simulink model "DisplayModel_Step3_done"  (R2013b)
settings: Solver=FixedStepDiscrete  StartTime=0.0  StopTime=10.0  FixedStep=0.2  RelTol=1e-3
undefined symbols (not defined in the file): sldvsubsys
libraries: simulink x6, sldvlib x3
settings Model: CovPath=LandingGearModes  CovMetricSettings=dcmw  CovHTMLOptions=-sRT=1 -aTS=1 -bRG=1 -bTC=1 -hTR=0 -nFC=0 -scm=1 -bcm=1 -xEv=0  CovModelRefEnable=off  Creator=siddhars  LastModifiedBy=rruff
settings OptimizationCC: InlineParams=on  ExpressionDepthLimit=2147483647  OptimizeModelRefInitCode=on  LifeSpan=1
settings DebuggingCC: StateNameClashWarn=warning
settings RTWCC: SystemTargetFile=ert.tlc  TemplateMakefile=ert_default_tmf  Description=Embedded Coder  ProcessScript=ert_make_rtw_hook  PortableWordSizes=on
settings CodeAppCC: IgnoreCustomStorageClasses=off  CustomSymbolStrType=$N$R$M  InternalIdentifier=Classic
settings ERTTargetCC: CodeReplacementLibrary=ANSI_C  GenerateSampleERTMain=on  InlinedParameterPlacement=NonHierarchical  ERTCustomFileTemplate=example_file_process.tlc
settings ConfigComp: Description=Design Verifier Custom Configuration Component  DVModelCoverageObjectives=MCDC  DVMaxTestCaseSteps=500  DVTestSuiteOptimization=CombinedObjectives (Nonlinear Extended)  DVSaveHarnessModel=on  DVModelReferenceHarness=on

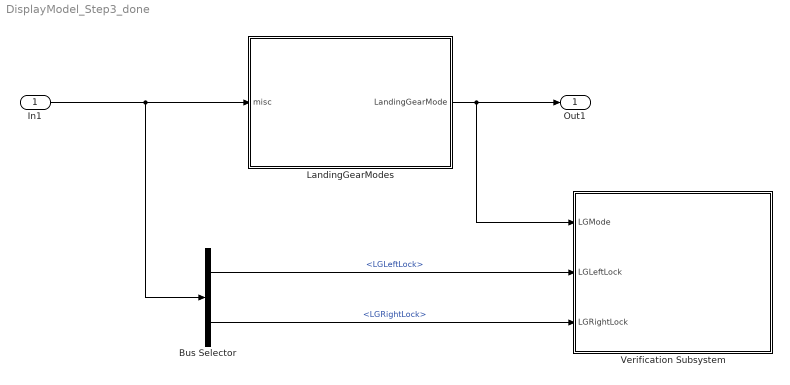
== system DisplayModel_Step3_done ==
  In1 : Inport  OutDataTypeStr=Bus: MiscData
  Bus Selector : BusSelector  OutputSignals=LGLeftLock,LGRightLock
  LandingGearModes : Stateflow chart  TreatAsAtomicUnit=on
  Verification Subsystem : Subsystem  Tag=VerificationSubsystem  DisableCoverage=on  LoadFcn=sldvsubsys('check')  TreatAsAtomicUnit=on  SimViewingDevice=on  mask(VerificationSubsystem){}
      mask init:
      | sldvsubsys('maskInit');
      settings: CopyFcn=sldvsubsys('copy');  OpenFcn=open_system(gcb,'force');
      settings: PreSaveFcn=|
      | set_param(gcb,'SimViewingDevice','on');
      | sldvsubsys('check');
      mask Help: helpview(fullfile(docroot,'toolbox','sldv','sldv.map'),'verificationsubsystem')
      mask Display: image(imread('sldvicon_versubsys.png','BackGroundColor',[1 1 1]),'center');
  Out1 : Outport
  wires:
  LandingGearModes/1(LandingGearMode) -> Out1/1, Verification Subsystem/1(LGMode)
  In1/1 -> LandingGearModes/1(misc), Bus Selector/1
  Bus Selector/1 -> Verification Subsystem/2(LGLeftLock)  "<LGLeftLock>"
  Bus Selector/2 -> Verification Subsystem/3(LGRightLock)  "<LGRightLock>"

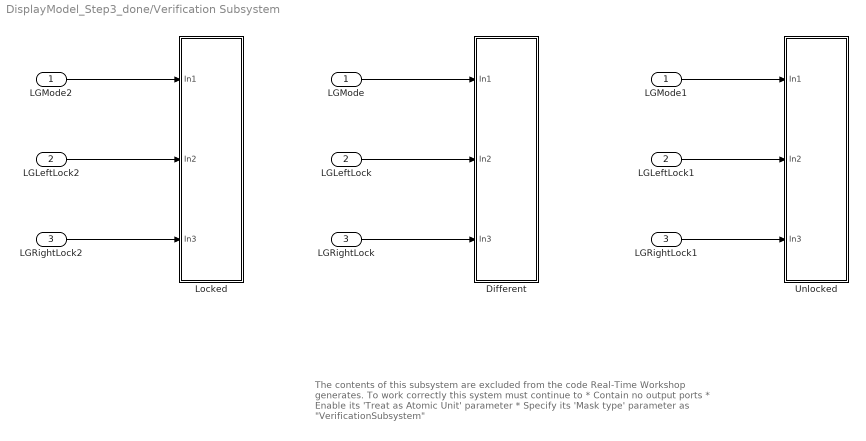
== system DisplayModel_Step3_done/Verification Subsystem ==
  note: The contents of this subsystem are excluded from the code Real-Time
      | Workshop generates.
      |
      | To work correctly this system must continue to
      | * Contain no output ports
      | * Enable its 'Treat as Atomic Unit' parameter
      | * Specify its 'Mask type' parameter as "VerificationSubsystem"
  LGMode : Inport
  LGLeftLock : Inport  Port=2
  LGRightLock : Inport  Port=3
  Different : Subsystem
  LGLeftLock1 : InportShadow  Port=2
  LGLeftLock2 : InportShadow  Port=2
  LGMode1 : InportShadow
  LGMode2 : InportShadow
  LGRightLock1 : InportShadow  Port=3
  LGRightLock2 : InportShadow  Port=3
  Locked : Subsystem
  Unlocked : Subsystem
  wires:
  LGMode2/1 -> Locked/1(In1)
  LGRightLock2/1 -> Locked/3(In3)
  LGLeftLock2/1 -> Locked/2(In2)
  LGMode/1 -> Different/1(In1)
  LGRightLock/1 -> Different/3(In3)
  LGLeftLock/1 -> Different/2(In2)
  LGMode1/1 -> Unlocked/1(In1)
  LGRightLock1/1 -> Unlocked/3(In3)
  LGLeftLock1/1 -> Unlocked/2(In2)

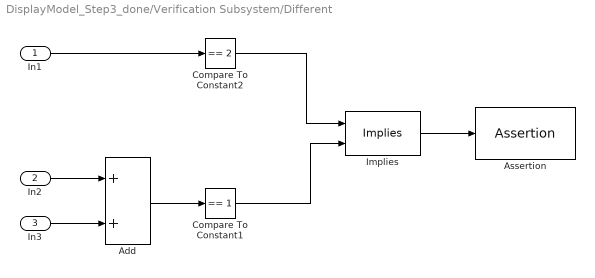
== system DisplayModel_Step3_done/Verification Subsystem/Different ==
  In1 : Inport
  In2 : Inport  Port=2
  In3 : Inport  Port=3
  Add : Sum
  Assertion : Assertion
  Compare To Constant1 : simulink/Logic and Bit Operations/Compare To Constant  relop===  const=1  OutDataTypeStr=uint8
  Compare To Constant2 : simulink/Logic and Bit Operations/Compare To Constant  relop===  const=2  OutDataTypeStr=boolean
  Implies : sldvlib/Verification Utilities/Implies
  wires:
  Implies/1 -> Assertion/1
  Compare To Constant2/1 -> Implies/1
  In1/1 -> Compare To Constant2/1
  Add/1 -> Compare To Constant1/1
  Compare To Constant1/1 -> Implies/2
  In2/1 -> Add/1
  In3/1 -> Add/2

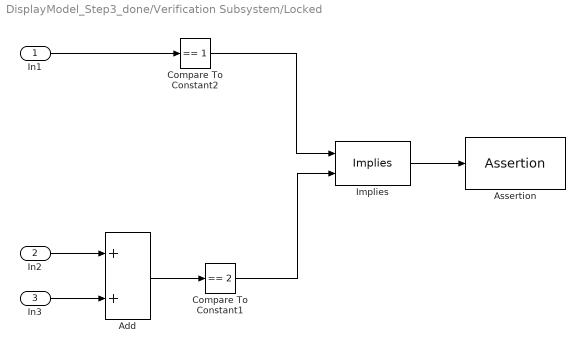
== system DisplayModel_Step3_done/Verification Subsystem/Locked ==
  In1 : Inport
  In2 : Inport  Port=2
  In3 : Inport  Port=3
  Add : Sum
  Assertion : Assertion
  Compare To Constant1 : simulink/Logic and Bit Operations/Compare To Constant  relop===  const=2  OutDataTypeStr=uint8
  Compare To Constant2 : simulink/Logic and Bit Operations/Compare To Constant  relop===  const=1  OutDataTypeStr=uint8
  Implies : sldvlib/Verification Utilities/Implies
  wires:
  Add/1 -> Compare To Constant1/1
  Implies/1 -> Assertion/1
  Compare To Constant2/1 -> Implies/1
  Compare To Constant1/1 -> Implies/2
  In1/1 -> Compare To Constant2/1
  In2/1 -> Add/1
  In3/1 -> Add/2

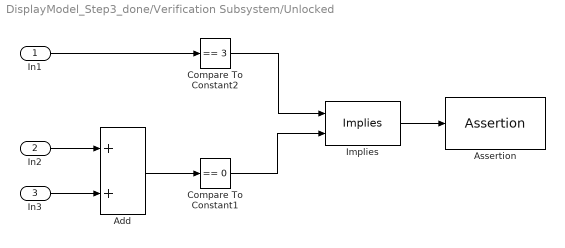
== system DisplayModel_Step3_done/Verification Subsystem/Unlocked ==
  In1 : Inport
  In2 : Inport  Port=2
  In3 : Inport  Port=3
  Add : Sum
  Assertion : Assertion
  Compare To Constant1 : simulink/Logic and Bit Operations/Compare To Constant  relop===  const=0  OutDataTypeStr=uint8
  Compare To Constant2 : simulink/Logic and Bit Operations/Compare To Constant  relop===  const=3  OutDataTypeStr=uint8
  Implies : sldvlib/Verification Utilities/Implies
  wires:
  Implies/1 -> Assertion/1
  Compare To Constant2/1 -> Implies/1
  In1/1 -> Compare To Constant2/1
  Add/1 -> Compare To Constant1/1
  Compare To Constant1/1 -> Implies/2
  In2/1 -> Add/1
  In3/1 -> Add/2

== stateflow chart DisplayModel_Step3_done/LandingGearModes ==
  state LeftLock [parallel]
    settings: executionOrder=1
    state Unlocked
    state Locked
    (default) -> (junction 122)
    (junction 122) -> LeftLock.Unlocked [order 2]
    (junction 122) -> LeftLock.Locked [order 1] : [misc.LGLeftLock]
    LeftLock.Locked -> LeftLock.Unlocked : [~misc.LGLeftLock]
    LeftLock.Unlocked -> LeftLock.Locked : [misc.LGLeftLock]
  state RightLock [parallel]
    settings: executionOrder=2
    state Unlocked
    state Locked
    (default) -> (junction 136)
    (junction 136) -> RightLock.Unlocked [order 2]
    (junction 136) -> RightLock.Locked [order 1] : [misc.LGRightLock]
    RightLock.Locked -> RightLock.Unlocked : [~misc.LGRightLock]
    RightLock.Unlocked -> RightLock.Locked : [misc.LGRightLock]
  state WarningModes [parallel]
    settings: executionOrder=3
    state BothLocked
      entry:
      LandingGearMode = 1;
    state BothUnLocked
      entry:
      LandingGearMode = 3;
    state OnlyOneLocked
      entry:
      LandingGearMode = 2;
    (default) -> (junction 102)
    (junction 102) -> BothLocked [order 1] : [in(LeftLock.Locked) &&...
        | in(RightLock.Locked)]
    (junction 102) -> BothUnLocked [order 2] : [in(LeftLock.Unlocked) &&...
        | in(RightLock.Unlocked)]
    (junction 102) -> OnlyOneLocked [order 3]
    BothUnLocked -> OnlyOneLocked [order 2] : [in(LeftLock.Locked) ||...
        | in(RightLock.Locked)]
    OnlyOneLocked -> BothLocked [order 2] : [in(LeftLock.Locked) &&...
        | in(RightLock.Locked)]
    OnlyOneLocked -> BothUnLocked [order 1] : [in(LeftLock.Unlocked) &&...
        | in(RightLock.Unlocked)]
    BothLocked -> OnlyOneLocked [order 2] : [in(LeftLock.Unlocked) ||...
        | in(RightLock.Unlocked)]
    BothLocked -> BothUnLocked [order 1] : [in(LeftLock.Unlocked) &&...
        | in(RightLock.Unlocked)]
    BothUnLocked -> BothLocked [order 1] : [in(LeftLock.Locked) &&...
        | in(RightLock.Locked)]
  data: misc input Bus: MiscData; LandingGearMode output double size=1
